simulink library "csc_kin_kinematic_propagation_lib"  (R2014b)
settings: Solver=ode45  StartTime=0.0  StopTime=10.0  RelTol=1e-3
undefined symbols (not defined in the file): ini_moon_rotation_rate, ini_tgt_landing_mcmf_pos
libraries: util_quat_lib x9, util_common_lib x3, util_frame_rotation_lib x2, util_info_lib x1
settings Model: Creator=escrane  LastModifiedBy=mstewart

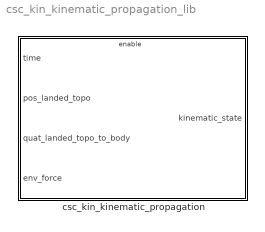
== system csc_kin_kinematic_propagation_lib ==
  csc_kin_kinematic_propagation : Subsystem

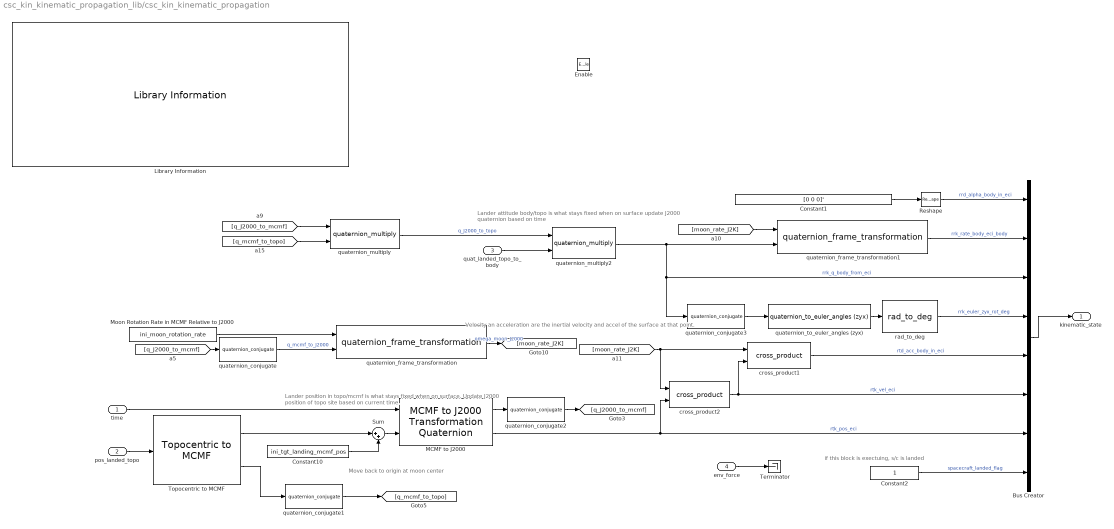
== system csc_kin_kinematic_propagation_lib/csc_kin_kinematic_propagation ==
  note: Velocity an acceleration are the inertial velocity and accel of the surface at that point.
  note: Lander position in topo/mcmf is what stays fixed when on surface.
      | Update J2000 position of topo site based on current time.
  note: Lander attitude body/topo is what stays fixed when on surface
      | update J2000 quaternion based on time
  note: Move back to origin at moon center
  note: if this block is exectuing, s/c is landed
  time : Inport
  pos_landed_topo : Inport  Port=2
  quat_landed_topo_to_body : Inport  Port=3
  env_force : Inport  Port=4
  Enable : EnablePort
  Bus Creator : BusCreator  Inputs=8  OutDataTypeStr=Bus: lander_state_bus_t
  Constant1 : Constant  Value=[0 0 0]'  VectorParams1D=off
  Constant10 : Constant  Value=ini_tgt_landing_mcmf_pos
  Constant2 : Constant
  Library Information : util_info_lib/Library Information  owner='escrane'
  "MCMF to J2000 " : util_frame_rotation_lib/MCMF to J2000  Transformation Quaternion
  Moon Rotation Rate in MCMF Relative to J2000 : Constant  Value=ini_moon_rotation_rate
  Reshape : Reshape
  Sum : Sum  Inputs=|++
  Terminator : Terminator
  Topocentric to MCMF : util_frame_rotation_lib/Topocentric to MCMF  SystemSampleTime=-1
  cross_product1 : util_common_lib/cross_product  SystemSampleTime=-1
  cross_product2 : util_common_lib/cross_product  SystemSampleTime=-1
  quaternion_conjugate{,1..3} (4 alike) : util_quat_lib/quaternion_conjugate  SystemSampleTime=-1
  quaternion_frame_transformation : util_quat_lib/quaternion_frame_transformation  SystemSampleTime=-1
  quaternion_frame_transformation1 : util_quat_lib/quaternion_frame_transformation  SystemSampleTime=-1
  quaternion_multiply : util_quat_lib/quaternion_multiply  SystemSampleTime=-1
  quaternion_multiply2 : util_quat_lib/quaternion_multiply  SystemSampleTime=-1
  quaternion_to_euler_angles (zyx) : util_quat_lib/quaternion_to_euler_angles (zyx)  SystemSampleTime=-1
  rad_to_deg : util_common_lib/rad_to_deg  SystemSampleTime=-1
  kinematic_state : Outport
  wires:
  Constant2/1 -> Bus Creator/8  "spacecraft_landed_flag"
  quaternion_conjugate3/1 -> quaternion_to_euler_angles (zyx)/1
  env_force/1 -> Terminator/1
  Sum/1 -> "MCMF to J2000 "/2
  Constant10/1 -> Sum/2
  Topocentric to MCMF/1 -> Sum/1
  [moon_rate_J2K] -> quaternion_frame_transformation1/1
  [moon_rate_J2K] -> cross_product2/1, cross_product1/1
  quaternion_frame_transformation/1 -> [moon_rate_J2K]  "omega_moon_J2000"
  [q_J2000_to_mcmf] -> quaternion_conjugate/1
  "MCMF to J2000 "/2 -> Bus Creator/7, cross_product2/2  "rtk_pos_eci"
  Moon Rotation Rate in MCMF Relative to J2000/1 -> quaternion_frame_transformation/1
  quaternion_conjugate/1 -> quaternion_frame_transformation/2  "q_mcmf_to_J2000"
  Constant1/1 -> Reshape/1
  cross_product2/1 -> Bus Creator/6, cross_product1/2  "rtk_vel_eci"
  cross_product1/1 -> Bus Creator/5  "rtd_acc_body_in_eci"
  quaternion_frame_transformation1/1 -> Bus Creator/2  "rrk_rate_body_eci_body"
  quaternion_to_euler_angles (zyx)/1 -> rad_to_deg/1
  rad_to_deg/1 -> Bus Creator/4  "rrk_euler_zyx_rot_deg"
  [q_J2000_to_mcmf] -> quaternion_multiply/1
  [q_mcmf_to_topo] -> quaternion_multiply/2
  quaternion_multiply/1 -> quaternion_multiply2/1  "q_J2000_to_topo"
  Reshape/1 -> Bus Creator/1  "rrd_alpha_body_in_eci"
  quat_landed_topo_to_body/1 -> quaternion_multiply2/2
  pos_landed_topo/1 -> Topocentric to MCMF/1
  time/1 -> "MCMF to J2000 "/1
  Topocentric to MCMF/2 -> quaternion_conjugate1/1
  quaternion_conjugate1/1 -> [q_mcmf_to_topo]
  "MCMF to J2000 "/1 -> quaternion_conjugate2/1
  quaternion_conjugate2/1 -> [q_J2000_to_mcmf]
  quaternion_multiply2/1 -> Bus Creator/3, quaternion_conjugate3/1, quaternion_frame_transformation1/2  "rrk_q_body_from_eci"
  Bus Creator/1 -> kinematic_state/1
